simulink model "S_PIL_BLOCK"  (R2017a)
settings: Solver=VariableStepAuto  StartTime=0.0  StopTime=10.0  RelTol=1e-3
libraries: pil_lib x1
settings Model: Creator=dricl  LastModifiedBy=dricl

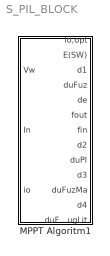
== system S_PIL_BLOCK ==
  MPPT Algoritm1 : Subsystem  DialogController=pil_create_dialog  LoadFcn=|
      | try
      |    if ~strcmp(rtw.pil.getPILVersion, '6.12 (R2017a)_12')
      |       set_param(gcb, 'DialogController', '');
      |       set_param(gcb, 'DialogControllerArgs', '');
      |    end
      | catch e
      |       set_param(gcb, 'DialogController', '');
      |       set_param(gcb, 'DialogControllerArgs', '');
      | end
      mask help: PIL:pil:XILBlockMaskDesc
      mask Display: disp('PIL');

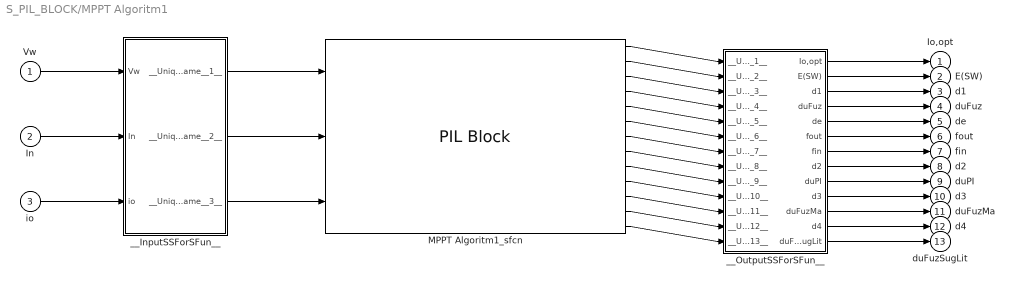
== system S_PIL_BLOCK/MPPT Algoritm1 ==
  Vw : Inport
  In : Inport  Port=2
  io : Inport  Port=3
  MPPT Algoritm1_sfcn : pil_lib/PIL Block  SimulationMode=PIL  IsTopModelPIL=off  CodeDir=C:\Users\dricl\OneDrive\Escritorio\Matlab_PIL_Journals\MPPT_ert_rtw  ConfigName=Texas Instruments C2000 Concerto Serial  XrelIsTopModelCode=on
  __InputSSForSFun__ : Subsystem
  __OutputSSForSFun__ : Subsystem
  Io,opt : Outport
  E(SW) : Outport  Port=2
  d1 : Outport  Port=3
  duFuz : Outport  Port=4
  de : Outport  Port=5
  fout : Outport  Port=6
  fin : Outport  Port=7
  d2 : Outport  Port=8
  duPI : Outport  Port=9
  d3 : Outport  Port=10
  duFuzMa : Outport  Port=11
  d4 : Outport  Port=12
  duFuzSugLit : Outport  Port=13
  wires:
  Vw/1 -> __InputSSForSFun__/1(Vw)
  In/1 -> __InputSSForSFun__/2(In)
  io/1 -> __InputSSForSFun__/3(io)
  __InputSSForSFun__/1(__UniqueOutportName__1__) -> MPPT Algoritm1_sfcn/1
  __InputSSForSFun__/2(__UniqueOutportName__2__) -> MPPT Algoritm1_sfcn/2
  __InputSSForSFun__/3(__UniqueOutportName__3__) -> MPPT Algoritm1_sfcn/3
  MPPT Algoritm1_sfcn/1 -> __OutputSSForSFun__/1(__UniqueInportName__1__)
  MPPT Algoritm1_sfcn/2 -> __OutputSSForSFun__/2(__UniqueInportName__2__)
  MPPT Algoritm1_sfcn/3 -> __OutputSSForSFun__/3(__UniqueInportName__3__)
  MPPT Algoritm1_sfcn/4 -> __OutputSSForSFun__/4(__UniqueInportName__4__)
  MPPT Algoritm1_sfcn/5 -> __OutputSSForSFun__/5(__UniqueInportName__5__)
  MPPT Algoritm1_sfcn/6 -> __OutputSSForSFun__/6(__UniqueInportName__6__)
  MPPT Algoritm1_sfcn/7 -> __OutputSSForSFun__/7(__UniqueInportName__7__)
  MPPT Algoritm1_sfcn/8 -> __OutputSSForSFun__/8(__UniqueInportName__8__)
  MPPT Algoritm1_sfcn/9 -> __OutputSSForSFun__/9(__UniqueInportName__9__)
  MPPT Algoritm1_sfcn/10 -> __OutputSSForSFun__/10(__UniqueInportName__10__)
  MPPT Algoritm1_sfcn/11 -> __OutputSSForSFun__/11(__UniqueInportName__11__)
  MPPT Algoritm1_sfcn/12 -> __OutputSSForSFun__/12(__UniqueInportName__12__)
  MPPT Algoritm1_sfcn/13 -> __OutputSSForSFun__/13(__UniqueInportName__13__)
  __OutputSSForSFun__/1(Io,opt) -> Io,opt/1
  __OutputSSForSFun__/2(E(SW)) -> E(SW)/1
  __OutputSSForSFun__/3(d1) -> d1/1
  __OutputSSForSFun__/4(duFuz) -> duFuz/1
  __OutputSSForSFun__/5(de) -> de/1
  __OutputSSForSFun__/6(fout) -> fout/1
  __OutputSSForSFun__/7(fin) -> fin/1
  __OutputSSForSFun__/8(d2) -> d2/1
  __OutputSSForSFun__/9(duPI) -> duPI/1
  __OutputSSForSFun__/10(d3) -> d3/1
  __OutputSSForSFun__/11(duFuzMa) -> duFuzMa/1
  __OutputSSForSFun__/12(d4) -> d4/1
  __OutputSSForSFun__/13(duFuzSugLit) -> duFuzSugLit/1

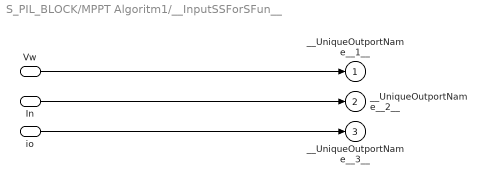
== system S_PIL_BLOCK/MPPT Algoritm1/__InputSSForSFun__ ==
  Vw : Inport
  In : Inport  Port=2
  io : Inport  Port=3
  __UniqueOutportName__1__ : Outport
  __UniqueOutportName__2__ : Outport  Port=2
  __UniqueOutportName__3__ : Outport  Port=3
  wires:
  Vw/1 -> __UniqueOutportName__1__/1
  In/1 -> __UniqueOutportName__2__/1
  io/1 -> __UniqueOutportName__3__/1

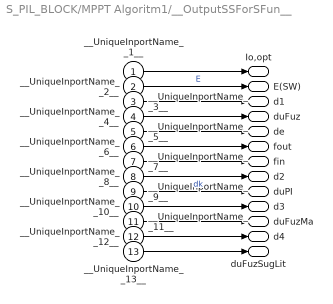
== system S_PIL_BLOCK/MPPT Algoritm1/__OutputSSForSFun__ ==
  __UniqueInportName__1__ : Inport
  __UniqueInportName__2__ : Inport  Port=2
  __UniqueInportName__3__ : Inport  Port=3
  __UniqueInportName__4__ : Inport  Port=4
  __UniqueInportName__5__ : Inport  Port=5
  __UniqueInportName__6__ : Inport  Port=6
  __UniqueInportName__7__ : Inport  Port=7
  __UniqueInportName__8__ : Inport  Port=8
  __UniqueInportName__9__ : Inport  Port=9
  __UniqueInportName__10__ : Inport  Port=10
  __UniqueInportName__11__ : Inport  Port=11
  __UniqueInportName__12__ : Inport  Port=12
  __UniqueInportName__13__ : Inport  Port=13
  Io,opt : Outport
  E(SW) : Outport  Port=2
  d1 : Outport  Port=3
  duFuz : Outport  Port=4
  de : Outport  Port=5
  fout : Outport  Port=6
  fin : Outport  Port=7
  d2 : Outport  Port=8
  duPI : Outport  Port=9
  d3 : Outport  Port=10
  duFuzMa : Outport  Port=11
  d4 : Outport  Port=12
  duFuzSugLit : Outport  Port=13
  wires:
  __UniqueInportName__1__/1 -> Io,opt/1
  __UniqueInportName__2__/1 -> E(SW)/1  "E"
  __UniqueInportName__3__/1 -> d1/1
  __UniqueInportName__4__/1 -> duFuz/1
  __UniqueInportName__5__/1 -> de/1
  __UniqueInportName__6__/1 -> fout/1
  __UniqueInportName__7__/1 -> fin/1
  __UniqueInportName__8__/1 -> d2/1
  __UniqueInportName__9__/1 -> duPI/1  "dk"
  __UniqueInportName__10__/1 -> d3/1
  __UniqueInportName__11__/1 -> duFuzMa/1
  __UniqueInportName__12__/1 -> d4/1
  __UniqueInportName__13__/1 -> duFuzSugLit/1
